simulink model "actions"  (R2017a)
settings: Solver=FixedStepDiscrete  StartTime=0.0  StopTime=30  FixedStep=0.1  RelTol=1e-3  EnableMultiTasking=on
undefined symbols (not defined in the file): sigbuilder_block
settings Model: NumberOfSteps=10  Creator=thr  LastModifiedBy=thr
settings SolverCC: AutoInsertRateTranBlk=on
settings DataIOCC: LimitDataPoints=on
settings OptimizationCC: LifeSpan=inf
settings DebuggingCC: AllowSymbolicDim=off  SFUnexpectedBacktrackingDiag=warning  SFNoUnconditionalDefaultTransitionDiag=warning  SFExecutionAtInitializationDiag=none
settings SFSimCC: SimCustomHeaderCode=|
  | #include "doubleIt.h"
  | #include "toBool.h"
settings SFSimCC: SimUserSources=|
  | doubleIt.c
  | toBool.c
settings GRTTargetCC: TargetLangStandard=C89/C90 (ANSI)  GeneratePreprocessorConditionals=Disable all
settings ConfigComp: CovMetricSettings=dw  CovHtmlReporting=on  CovSaveCumulativeToWorkspaceVar=on  CovSaveSingleToWorkspaceVar=on  CovShowResultsExplorer=off  CovExternalEMLEnable=off  CovSFcnEnable=off

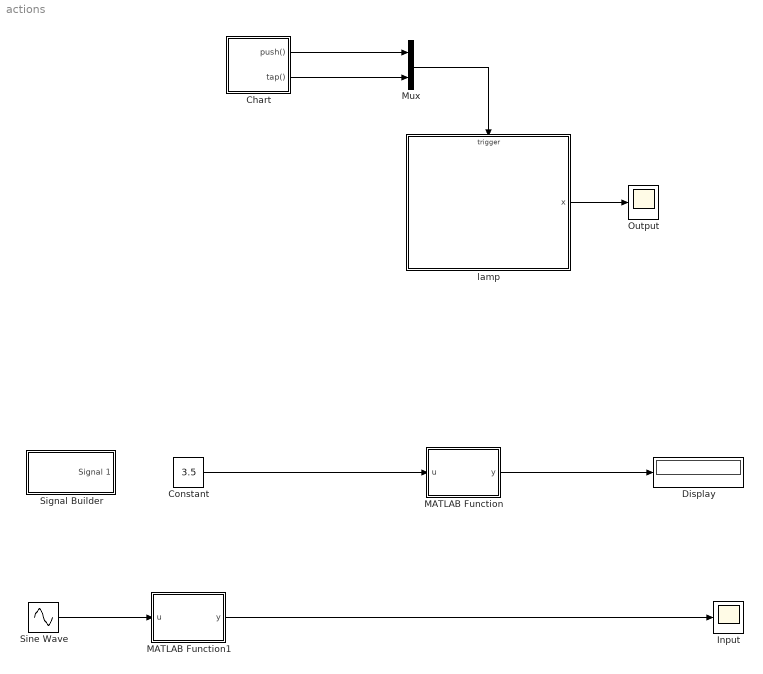
== system actions ==
  Chart : Stateflow chart  TreatAsAtomicUnit=on
  Constant : Constant  Value=3.5
  Display : Display
  Input : Scope
  MATLAB Function : MATLAB Function  TreatAsAtomicUnit=on
  MATLAB Function1 : MATLAB Function  TreatAsAtomicUnit=on
  Mux : Mux  Inputs=2
  Output : Scope
  Signal Builder : Subsystem  Tag=STV Subsys  LoadFcn=sigbuilder_block('load');  StartFcn=sigbuilder_block('start');  StopFcn=sigbuilder_block('stop');  ClipboardFcn=sigbuilder_block('clipboard');  mask(Sigbuilder block){tuvar=[0:10]}
      mask help: Simulink:masks:SigbuilderBlock_MD
      mask init:
      | if ~strcmp(get_param(bdroot(gcbh),'SimulationStatus'),'stopped') tuvar = sigbuilder_block('maskInit'); end
      settings: CopyFcn=sigbuilder_block('copy');  DeleteFcn=sigbuilder_block('delete');  ModelCloseFcn=sigbuilder_block('modelClose');  PreSaveFcn=sigbuilder_block('preSave');  PauseFcn=sigbuilder_block('pause');  ContinueFcn=sigbuilder_block('continue');  NameChangeFcn=sigbuilder_block('namechange');  OpenFcn=sigbuilder_block('open',[437.6 199.2 550.4 400 ]);  CloseFcn=sigbuilder_block('close');
      mask Display: plot(0, 0, 100, 100,[2, 2, 32, 32, 2], [68, 8, 8, 68, 68],[32, 2], [38, 38], [32, 19, 2],[53, 60, 44], [32, 17, 17, 2],[16, 16, 31, 31]);txt = getActiveGroup(gcbh);text(2, 100, txt,'verticalAlignment', 'top');
  Sine Wave : Sin  Amplitude=3  SampleTime=0
  lamp : Stateflow chart  TreatAsAtomicUnit=on
  wires:
  Constant/1 -> MATLAB Function/1(u)
  MATLAB Function/1(y) -> Display/1
  Sine Wave/1 -> MATLAB Function1/1(u)
  MATLAB Function1/1(y) -> Input/1
  lamp/1(x) -> Output/1
  Mux/1 -> lamp/Trigger
  Chart/1(push()) -> Mux/1
  Chart/2(tap()) -> Mux/2

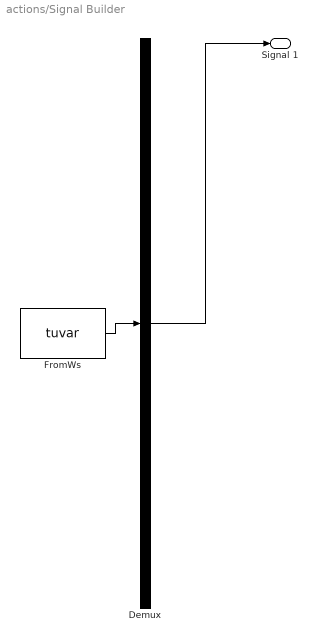
== system actions/Signal Builder ==
  Demux : Demux  Tag=STV Demux  Outputs=1
  FromWs : FromWorkspace  Tag=STV FromWs  VariableName=tuvar  SampleTime=0
      SigBuilderData=|
      | common.afterFinalStr = 'Extrapolate'
      | common.sampleTime = 0
      | dataSet.timeRange = [0 10]
      | dataSet.name = 'Group 1'
      | sbobj.Groups.Name = 'Group 1'
      | sbobj.Groups.Signals.Name = 'Signal 1'
      | sbobj.Groups.Signals.XData = [0 4 4 6 6 10]
      | sbobj.Groups.Signals.YData = [0 0 1 1 0 0]
  Signal 1 : Outport  Tag=STV Outport
  wires:
  Demux/1 -> Signal 1/1
  FromWs/1 -> Demux/1

== matlab function actions/MATLAB Function1 ==
  data: u input; y output
function y = convertToBool(u)

y = false;
y = coder.ceval('toBool',u);

== matlab function actions/MATLAB Function ==
  data: u input; y output
function y = callingDoubleIt(u)

y = 0.0;
y = coder.ceval('doubleIt',u);

== stateflow chart actions/lamp ==
  settings: executeAtInitialization=1
  state S1
    entry: x = 2
  state S2
    exit: x = 3
  state S3
  state S4
    during: x = 4
  state S5
  (default) -> S1
  S3 -> S4 : push
  S2 -> S3 [order 1] : push
  S1 -> S2 : push
  S2 -> S5 [order 2] : tap
  data: x output int32
  events: push input FUNCTION_CALL_EVENT; tap input FUNCTION_CALL_EVENT

== stateflow chart actions/Chart ==
  state A
    entry: c = c + 1
  (default) -> A : {c=1}
  A -> A [order 2] : after(2, sec){push}
  A -> A [order 1] : [c==30]{tap}
  data: c local
  events: push output FUNCTION_CALL_EVENT; tap output FUNCTION_CALL_EVENT
